simulink model "ex02"  (R2022b)
settings: Solver=VariableStepAuto  StartTime=0.0  StopTime=600  RelTol=1e-3
settings Model: Creator=ACER  LastModifiedBy=ACER

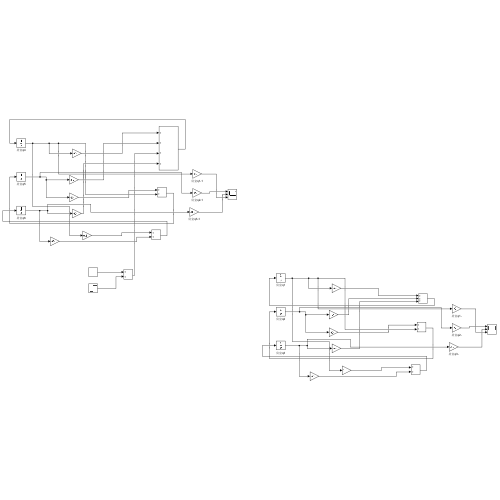
[thumbnail: Simulink's stored preview of the top-level diagram]
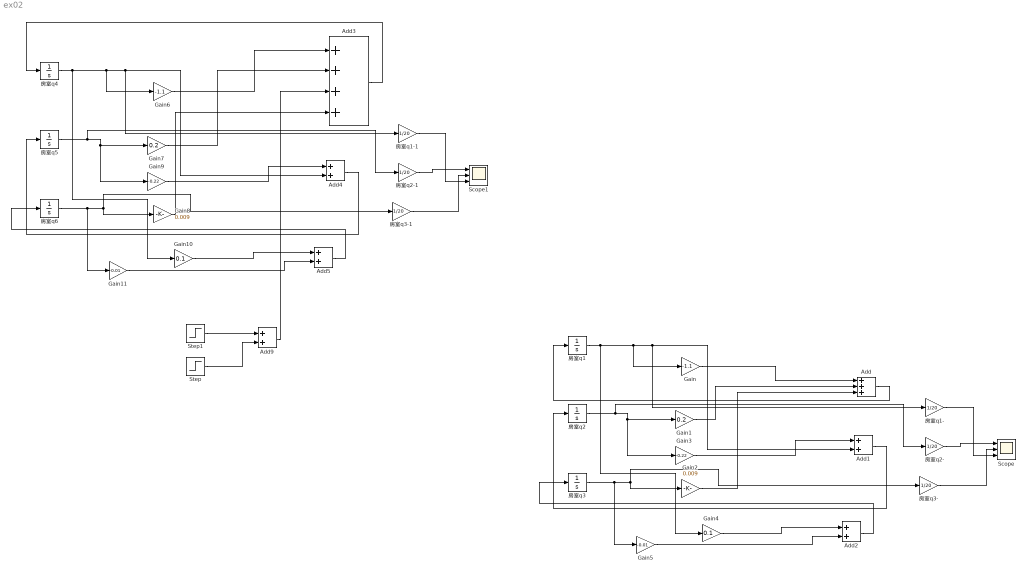
== system ex02 ==
  Add : Sum  Inputs=+++
  Add{1..2,4..5,9} (5 alike) : Sum
  Add3 : Sum  Inputs=++++
  Gain : Gain  Gain=-1.1
  Gain1 : Gain  Gain=0.2
  Gain10 : Gain  Gain=0.1
  Gain11 : Gain  Gain=-0.01
  Gain2 : Gain  Gain=0.009
  Gain3 : Gain  Gain=-0.22
  Gain4 : Gain  Gain=0.1
  Gain5 : Gain  Gain=-0.01
  Gain6 : Gain  Gain=-1.1
  Gain7 : Gain  Gain=0.2
  Gain8 : Gain  Gain=0.009
  Gain9 : Gain  Gain=-0.22
  Scope : Scope  NumInputPorts=3
  Scope1 : Scope  NumInputPorts=3
  Step : Step  Time=0  SampleTime=0
  Step1 : Step  Time=20  After=-1  SampleTime=0
  房室q1 : Integrator  InitialCondition=1
  房室q1- : Gain  Gain=1/20
  房室q1-1 : Gain  Gain=1/20
  房室q{2..3,5..6} (4 alike) : Integrator
  房室q2- : Gain  Gain=1/20
  房室q2-1 : Gain  Gain=1/20
  房室q3- : Gain  Gain=1/20
  房室q3-1 : Gain  Gain=1/20
  房室q4 : Integrator  InitialCondition=1
  wires:
  房室q1/1 -> Gain4/1, 房室q1-/1, Add1/2, Gain/1
  Gain/1 -> Add/1
  房室q2/1 -> 房室q2-/1, Gain3/1, Gain1/1
  Gain1/1 -> Add/2
  房室q3/1 -> Gain5/1, Gain2/1, 房室q3-/1
  Gain2/1 -> Add/3
  Add/1 -> 房室q1/1
  Gain3/1 -> Add1/1
  Add1/1 -> 房室q2/1
  Gain4/1 -> Add2/1
  Gain5/1 -> Add2/2
  Add2/1 -> 房室q3/1
  房室q1-/1 -> Scope/3
  房室q2-/1 -> Scope/1
  房室q3-/1 -> Scope/2
  房室q3-1/1 -> Scope1/2
  Gain11/1 -> Add5/2
  房室q6/1 -> Gain11/1, Gain8/1, 房室q3-1/1
  Gain9/1 -> Add4/1
  房室q1-1/1 -> Scope1/3
  Gain8/1 -> Add3/4
  Gain10/1 -> Add5/1
  Add4/1 -> 房室q5/1
  Add5/1 -> 房室q6/1
  房室q2-1/1 -> Scope1/1
  Gain6/1 -> Add3/1
  房室q4/1 -> Gain10/1, 房室q1-1/1, Add4/2, Gain6/1
  Add3/1 -> 房室q4/1
  房室q5/1 -> 房室q2-1/1, Gain9/1, Gain7/1
  Gain7/1 -> Add3/2
  Step/1 -> Add9/2
  Step1/1 -> Add9/1
  Add9/1 -> Add3/3
